simulink model "modelo"  (R2013a)
settings: Solver=ode45  StartTime=0.0  StopTime=2  RelTol=1e-3
libraries: cstblocks x4, simulink x1
settings Model: Creator=Guilherme  LastModifiedBy=Guilherme

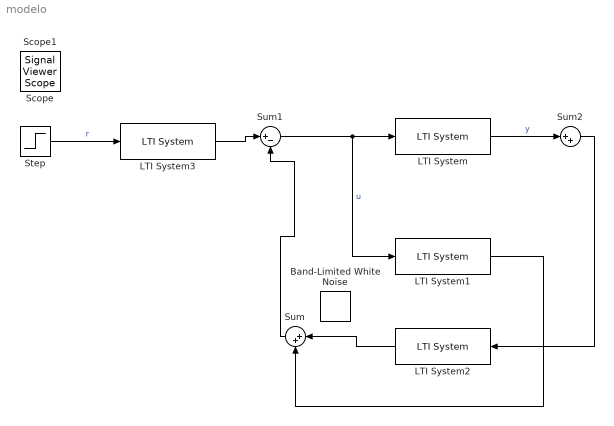
== system modelo ==
  LTI System : cstblocks/LTI System  sys=G  IC=[]
  LTI System1 : cstblocks/LTI System  sys=C_u  IC=[]
  LTI System2 : cstblocks/LTI System  sys=C_y  IC=[]
  LTI System3 : cstblocks/LTI System  sys=H  IC=[]
  Step : Step  Time=0  SampleTime=0
  Sum : Sum  Inputs=|++
  Sum1 : Sum  Inputs=|+-
  Sum2 : Sum  Inputs=|++
  Band-Limited White Noise : simulink/Sources/Band-Limited White Noise  IOType=siggen  Cov=1e-6  Ts=1e-3  seed=[23341]
  Scope : SignalViewerScope  IOType=viewer  RefreshTime=0.035000
  Scope1 : SignalViewerScope  IOType=viewer  NumInputPorts=2  RefreshTime=0.035000
      settings: YMin=-5~-5  YMax=5~5
  wires:
  LTI System3/1 -> Sum1/1
  Sum1/1 -> LTI System1/1, LTI System/1  "u"
  LTI System/1 -> Sum2/1  "y"
  LTI System1/1 -> Sum/2
  LTI System2/1 -> Sum/1
  Sum/1 -> Sum1/2
  Step/1 -> LTI System3/1  "r"
  Sum2/1 -> LTI System2/1
